simulink model "Bouncingcode"  (R2018b)
settings: Solver=VariableStepAuto  StartTime=0.0  StopTime=1000000000  RelTol=1e-3
libraries: vrlib x2
settings Model: Creator=Notebook  LastModifiedBy=Notebook

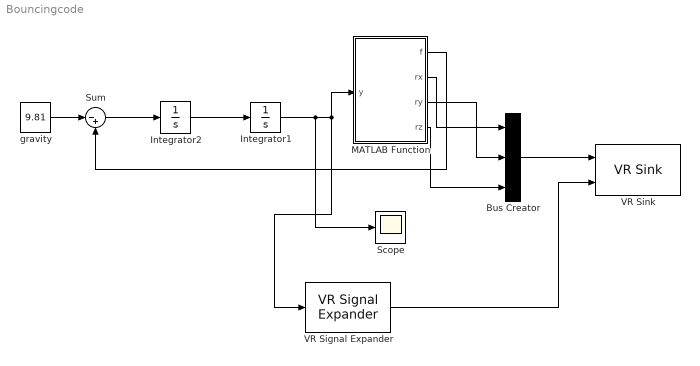
== system Bouncingcode ==
  Bus Creator : BusCreator  Inputs=3
  Integrator1 : Integrator  InitialCondition=20
  Integrator2 : Integrator
  MATLAB Function : MATLAB Function  TreatAsAtomicUnit=on
  Scope : Scope
  Sum : Sum  Inputs=|-+
  VR Signal Expander : vrlib/VR Signal Expander  outwidth=3  outidx=[2]
      settings: SourceProductName=Simulink 3D Animation  SourceProductBaseCode=VR
  VR Sink : vrlib/VR Sink  InstantiateOnLoad=on  SampleTime=0.01  ViewEnable=on  RemoteChange=off  RemoteView=on  FieldsWritten=Ball.scale.3.1.1.double#Ball.translation.3.1.1.double  WorldFileName=Bouncingcodenew.wrl  AutoView=off  VideoDimensions=[]  AllowVariableSize=off
      settings: SourceProductBaseCode=VR
  gravity : Constant  Value=9.81
  wires:
  gravity/1 -> Sum/1
  Sum/1 -> Integrator2/1
  Integrator2/1 -> Integrator1/1
  MATLAB Function/1(f) -> Sum/2
  Integrator1/1 -> Scope/1, VR Signal Expander/1, MATLAB Function/1(y)
  VR Signal Expander/1 -> VR Sink/2
  Bus Creator/1 -> VR Sink/1
  MATLAB Function/2(rx) -> Bus Creator/1
  MATLAB Function/3(ry) -> Bus Creator/2
  MATLAB Function/4(rz) -> Bus Creator/3

== matlab function Bouncingcode/MATLAB Function ==
  data: y input; f output; rx output; ry output; rz output
function [f,rx,ry,rz] = fcn(y)
if y<1e-4
    y=1e-4;
end
if y>=1.5
    f=0;
    rx=1.5;
    ry=1.5;
    rz=1.5;
else
    f=500*(1.5-y);
    rx=sqrt(1.5^3/y);
    ry=y;
    rz=rx;
end
